simulink model "TemplateForQ2"  (R2018b)
settings: Solver=VariableStepAuto  StartTime=0.0  StopTime=500e-3  RelTol=1e-3
libraries: powerlib x8, pePowerMeasurement x2
settings Model: Creator=Furkan  LastModifiedBy=MUHAMMED
settings DebuggingCC: LibraryContextMissingDiagnostic=none
settings SFSimCC: SimUseLocalCustomCode=off
settings RTWCC: RTWUseLocalCustomCode=off

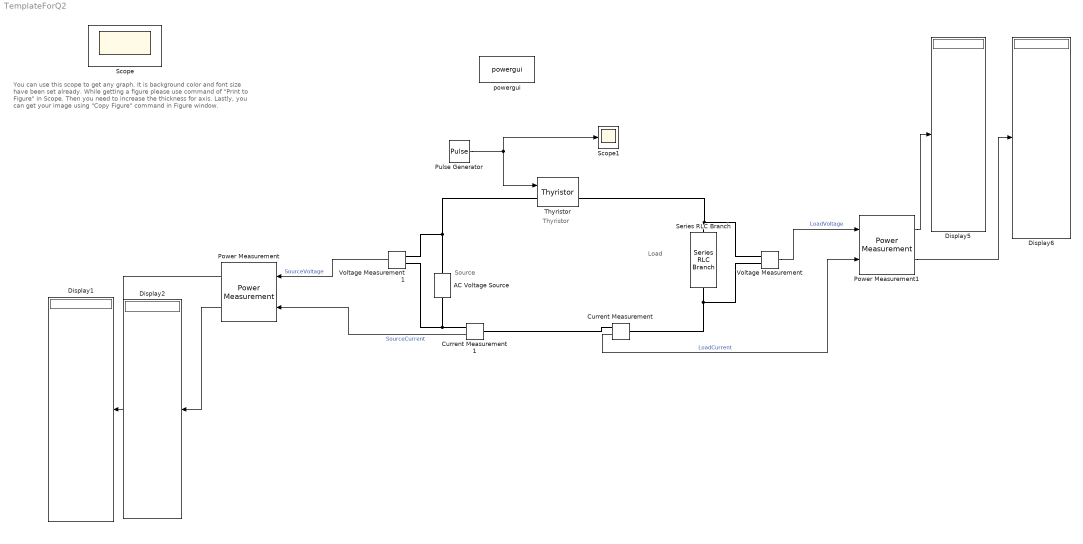
== system TemplateForQ2 ==
  note: You can use this scope to get any graph. It is background color and font size have been set already. While getting a figure please use command of "Print to Figure" in Scope. Then you need to increase the thickness for axis. Lastly, you can get your image using "Copy Figure" command in Figure window.
  note: Source
  note: Thyristor
  note: Load
  AC Voltage Source : powerlib/Electrical Sources/AC Voltage Source  Amplitude=325  Phase=0  Frequency=50  SampleTime=0  Measurements=None  BusType=swing  Pref=10e3  Qref=0  Qmin=-inf  Qmax=+inf
      settings: SourceProductName=Simscape Electrical
  Current Measurement : powerlib/Measurements/Current Measurement  PhasorSimulation=off  OutputType=Complex  PSBequivalent=0
      settings: SourceProductName=Simscape Electrical
  Current Measurement1 : powerlib/Measurements/Current Measurement  PhasorSimulation=off  OutputType=Complex  PSBequivalent=0
      settings: SourceProductName=Simscape Electrical
  Display{1..2,5..6} (4 alike) : Display
  Power Measurement : pePowerMeasurement/Power Measurement  LabelModeActiveChoice=Continuous  F=50  K=[0 1 2 3 4 5 6 7 8 9]  Ts=0
  Power Measurement1 : pePowerMeasurement/Power Measurement  LabelModeActiveChoice=Continuous  F=50  K=[0 1 2 3 4 5 6 7 8 9]  Ts=0
  Pulse Generator : DiscretePulseGenerator  PulseType=Time based  Period=20e-3  PulseWidth=5  PhaseDelay=5e-3
  Scope : Scope  NumInputPorts=4
  Scope1 : Scope
  Series RLC Branch : powerlib/Elements/Series RLC Branch  LConnTagsString=__new0  RConnTagsString=__new0  BranchType=RLC  Resistance=10  Inductance=0.01  SetiL0=off  InitialCurrent=0  Capacitance=0  Setx0=off  InitialVoltage=0  Measurements=None
      settings: SourceProductName=Simscape Electrical
  Thyristor : powerlib/Power Electronics/Thyristor  Ron=0.001  Lon=0  Vf=0.8  IC=0  Rs=500  Cs=250e-9  Measurements=on
      settings: SourceProductName=Simscape Electrical
  Voltage Measurement : powerlib/Measurements/Voltage Measurement  PhasorSimulation=off  OutputType=Complex  PSBequivalent=0
      settings: SourceProductName=Simscape Electrical
  Voltage Measurement1 : powerlib/Measurements/Voltage Measurement  PhasorSimulation=off  OutputType=Complex  PSBequivalent=0
      settings: SourceProductName=Simscape Electrical
  powergui : powerlib/powergui  Priority=1  SimulationMode=Continuous  SampleTime=50e-6  frequency=60  Iterations=50  frequencyindice=50  Pbase=100e6  ErrMax=1e-4  UnitsV=kV  UnitsW=MW  buscounter=0  FunctionMessages=off  echomessages=off  EnableUseOfTLC=off  CurrentSourceSwitches=off  DisableSnubberDevices=off  DisableRonSwitches=off  DisableVfSwitches=off  DisplayEquations=off  SolverType=Tustin/Backward Euler (TBE)  Interpol=off  ExternalGateDelay=off  methode=off  Ts=100  x0status=blocks  SPID=on  SwTol=0  HookPort=off  RestoreLinks=warning  ResistiveCurrentMeasurement=off  Frange=[0:2:500]  Ylog=off  Xlog=on  ShowGrid=off  save=off  variable=ZData  structure=Vs  ZoomFFT=off  StartTime=0.0  cycles=1  DisplayStyle=2  fundamental=50  FreqAxis=off  MaxFrequency=1000  frequencyindicesteady=1  RmsSteady=1  display=off
      settings: SourceProductName=Simscape Electrical
  wires:
  Voltage Measurement/1 -> Power Measurement1/1  "LoadVoltage"
  Power Measurement/1 -> Display1/1
  Power Measurement/2 -> Display2/1
  Power Measurement1/1 -> Display5/1
  Power Measurement1/2 -> Display6/1
  Pulse Generator/1 -> Scope1/1, Thyristor/1
  Voltage Measurement1/1 -> Power Measurement/1  "SourceVoltage"
  Current Measurement1/1 -> Power Measurement/2  "SourceCurrent"
  Current Measurement/1 -> Power Measurement1/2  "LoadCurrent"
  connections:
  Voltage Measurement/LConn1 -- Series RLC Branch/LConn1 -- Thyristor/RConn1
  Voltage Measurement1/LConn1 -- Thyristor/LConn1 -- AC Voltage Source/RConn1
  Voltage Measurement/LConn2 -- Current Measurement/LConn1 -- Series RLC Branch/RConn1
  Current Measurement1/RConn1 -- AC Voltage Source/LConn1 -- Voltage Measurement1/LConn2
  Current Measurement/RConn1 -- Current Measurement1/LConn1
